simulink model "LQRcontrol"  (R2018b)
settings: Solver=FixedStepAuto  StartTime=0.0  StopTime=20  FixedStep=0.00001  MaxStep=0.00001  RelTol=1e-3  EnableMultiTasking=on
InitFcn:
  | L = 0.4125 ; % Henry
  | Rl = 10 ; % ohm
  | Rs = 1 ; % ohm
  | Kf = 32654e-9 ; % N*m^2/Amp^2
  | g = 9810e-3 ; % m/sec^2 ;
  | m = 0.068 ; % kg
  | 
  | 
  | Yss = 0.01 ;
  | Iss = Yss * (m*g/Kf)^0.5 ;
  | Vss = Iss * (Rl  + Rs) ;
  | 
StopFcn:
  | figure(1) ;
  | subplot(211) ;
  | out.signals.values(: , 2) = 1e3*out.signals.values(: , 2) ;
  | plot(out.time  ,     out.signals.values(: , [1,2]) , 'LineWidth' , 2) ;
  | grid on
  | xlabel('Time   (Second)') ;
  | ylabel('Current  , Position') ;
  | legend('Current(Amp)','Position(mm)') ;
  | 
  | subplot(212) ;
  | plot(out.time  ,     out.signals.values(: , 4) , 'LineWidth' , 2) ;
  | grid on
  | xlabel('Time   (Second)') ;
  | ylabel('Voltage') ;
  | legend('Voltage') ;
values from neighbouring files (symbols this model uses):
  K = lqr(A , B , Q , R , N)    [DesignController.m]    (also in TrainNN.m = zeros(N, 3))
settings Model: Creator=omid_zandi  LastModifiedBy=lenovo
settings OptimizationCC: LifeSpan=inf
settings DebuggingCC: SFUnexpectedBacktrackingDiag=warning  SFNoUnconditionalDefaultTransitionDiag=warning
settings SFSimCC: SimUseLocalCustomCode=off
settings RTWCC: RTWUseLocalCustomCode=off
settings CodeAppCC: StateflowObjectComments=on
settings GRTTargetCC: TargetLangStandard=C89/C90 (ANSI)  GeneratePreprocessorConditionals=Disable all
settings ConfigComp: CovMetricSettings=dw  CovHtmlReporting=on  CovSaveCumulativeToWorkspaceVar=on  CovSaveSingleToWorkspaceVar=on  CovExternalEMLEnable=off

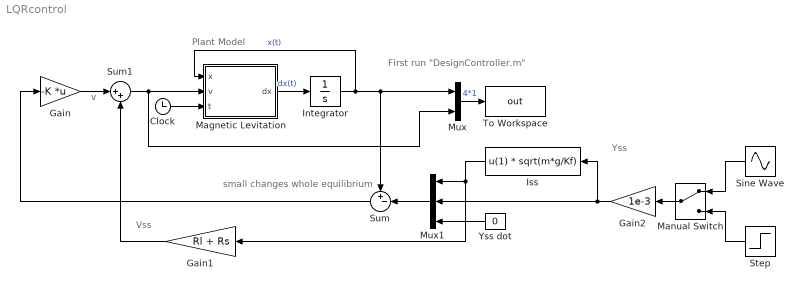
== system LQRcontrol ==
  note: First run "DesignController.m"
  note: Yss
  note: small changes whole equilibrium
  note: Vss
  note: Plant Model
  note: v
  Clock : Clock
  Gain : Gain  Gain=-K  Multiplication=Matrix(K*u)
  Gain1 : Gain  Gain=Rl + Rs
  Gain2 : Gain  Gain=1e-3
  Integrator : Integrator  InitialCondition=[Iss; Yss ; 0]
  "Iss " : Fcn  Expr=u(1) * sqrt(m*g/Kf)
  Magnetic Levitation : MATLAB Function  TreatAsAtomicUnit=on
  Manual Switch : ManualSwitch
  Mux : Mux  Inputs=2
  Mux1 : Mux  Inputs=3
  Sine Wave : Sin  Amplitude=10  Bias=20  Frequency=2*pi*0.05 %T = 20 second  SampleTime=0
  Step : Step  Time=10  Before=20  After=25  SampleTime=0
  Sum : Sum  Inputs=+-|
  Sum1 : Sum  Inputs=|++
  To Workspace : ToWorkspace  VariableName=out  SaveFormat=Structure With Time  SampleTime=-1
  Yss dot : Constant  Value=0
  wires:
  Integrator/1 -> Mux/1, Sum/1, Magnetic Levitation/1(x)  "x(t)"
  Magnetic Levitation/1(dx) -> Integrator/1  "dx(t)"
  Mux/1 -> To Workspace/1  "4*1"
  Clock/1 -> Magnetic Levitation/3(t)
  Mux1/1 -> Sum/2
  Gain2/1 -> "Iss "/1, Mux1/2
  "Iss "/1 -> Gain1/1, Mux1/1
  Yss dot/1 -> Mux1/3
  Sum/1 -> Gain/1
  Gain/1 -> Sum1/1
  Gain1/1 -> Sum1/2
  Sum1/1 -> Mux/2, Magnetic Levitation/2(v)
  Manual Switch/1 -> Gain2/1
  Sine Wave/1 -> Manual Switch/1
  Step/1 -> Manual Switch/2

== matlab function LQRcontrol/Magnetic Levitation ==
  data: x input; dx output; v input; t input
function dx = Model(x  , v, t)

L = 0.4125 ; % Henry
Rl = 10 ; % ohm
Rs = 1 ; % ohm
Kf = 32654e-9 ; % N*m^2/Amp^2
g = 9810e-3 ; % m/sec^2 ;
m = 0.068 ; % kg

F = 0.1*(t>=5)*(t <= 5.001) ; 
dx = zeros(3,1) ;
dx(1) = -(Rl + Rs)/L * x(1) + 1/L*v ;
dx(2) = x(3) ;
dx(3) = g + F/m - Kf/m*(x(1)/x(2))^2;
